simulink model "Avg_Arr"  (R2021a)
settings: Solver=FixedStepDiscrete  StartTime=0.0  StopTime=10.0  RelTol=1e-3
settings Model: Creator=Mohamed Elomda  LastModifiedBy=Mohamed Elomda

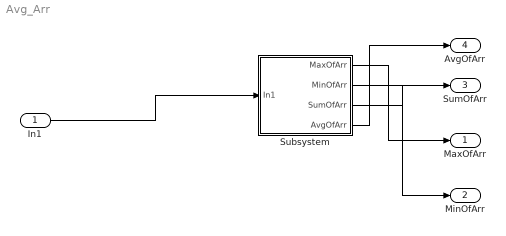
== system Avg_Arr ==
  In1 : Inport  PortDimensions=10
  Subsystem : Subsystem
  MaxOfArr : Outport
  MinOfArr : Outport  Port=2
  SumOfArr : Outport  Port=3
  AvgOfArr : Outport  Port=4
  wires:
  Subsystem/4(AvgOfArr) -> AvgOfArr/1
  Subsystem/2(MinOfArr) -> MinOfArr/1
  In1/1 -> Subsystem/1(In1)
  Subsystem/3(SumOfArr) -> SumOfArr/1
  Subsystem/1(MaxOfArr) -> MaxOfArr/1

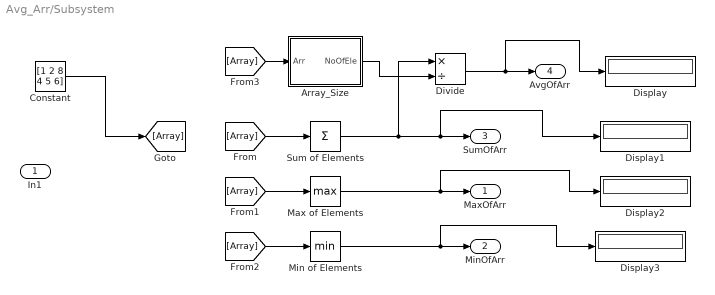
== system Avg_Arr/Subsystem ==
  In1 : Inport  PortDimensions=10
  Array_Size : MATLAB Function  TreatAsAtomicUnit=on
  Constant : Constant  Value=[1 2 8 4 5 6]
  Display{,1..3} (4 alike) : Display
  Divide : Product  Inputs=*/
  Max of Elements : MinMax  Function=max
  Min of Elements : MinMax
  Sum of Elements : Sum  Inputs=+
  MaxOfArr : Outport
  MinOfArr : Outport  Port=2
  SumOfArr : Outport  Port=3
  AvgOfArr : Outport  Port=4
  wires:
  [Array] -> Sum of Elements/1
  Array_Size/1(NoOfEle) -> Divide/2
  Divide/1 -> AvgOfArr/1, Display/1
  Sum of Elements/1 -> SumOfArr/1, Display1/1, Divide/1
  [Array] -> Array_Size/1(Arr)
  Max of Elements/1 -> MaxOfArr/1, Display2/1
  [Array] -> Max of Elements/1
  Constant/1 -> [Array]
  [Array] -> Min of Elements/1
  Min of Elements/1 -> MinOfArr/1, Display3/1

== matlab function Avg_Arr/Subsystem/Array_Size ==
  data: Arr input; NoOfEle output
function NoOfEle = fcn(Arr)
    NoOfEle = length(Arr);
